simulink model "TaskServiceBase_FSM_revB"  (R2015b)
settings: Solver=ode4  StartTime=0.0  StopTime=inf  FixedStep=.01  RelTol=1e-3
settings Model: Creator=elliocm  LastModifiedBy=elliocm

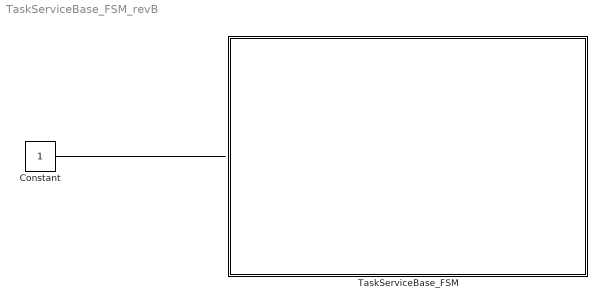
== system TaskServiceBase_FSM_revB ==
  Constant : Constant
  TaskServiceBase_FSM : Stateflow chart  RequirementInfo="{}  %GIDa_69d87331_3a4c_4800_b6a9_49c4bb62fd68"  TreatAsAtomicUnit=on
  wires:
  Constant/1 -> ?

== stateflow chart TaskServiceBase_FSM_revB/TaskServiceBase_FSM ==
  state Idle
    entry: state = 2
    state Idle_Request
      entry: SensorFootprintRequests_out = 0
    note: Simple Delay
        | (Consider Random Fail on TaskInit)
    state Idle_Success
      entry: SensorFootprintRequests_out = 1
    (default) -> Idle_Request
    Idle_Request -> (junction 51)
    (junction 51) -> Idle_Success : after(5,sec)
  state SensorRequest
    entry: state = 3
    state SensorRequest_Init
      entry: RouteRequest_out = 0
    note: Simple Delay
        | (Consider Random Fail on TaskInit)
    state SensorRequest_Success
      entry: RouteRequest_out = 1
    (default) -> SensorRequest_Init
    SensorRequest_Init -> (junction 64)
    (junction 64) -> SensorRequest_Success : after(3,sec)
  state Init
    entry: state = 1
    note: Simple Delay
        | (Consider Random Fail on TaskInit)
    state Init_Request
      entry: init_complete = 0
      TaskInitialized_out = 0
    state Init_Success
      entry: init_complete = 1
      TaskInitialized_out = 1
    (default) -> Init_Request
    Init_Request -> (junction 40)
    (junction 40) -> Init_Success : after(3,sec)
  state OptionRoutes
    entry: state = 4
    state OptionRoutes_Init
      entry: TaskPlanOptions_out = 0
    note: Simple Delay
        | (Consider Random Fail on TaskInit)
    state OptionRoutes_Success
      entry: TaskPlanOptions_out = 1
    (default) -> OptionRoutes_Init
    OptionRoutes_Init -> (junction 71)
    (junction 71) -> OptionRoutes_Success : after(10,sec)
  state Active
    entry: state = 8
    state Active_Init
      entry: TaskComplete_out = 0
    note: Simple Delay
        | (Consider Random Fail on TaskInit)
    state Active_Success
      entry: TaskComplete_out = 1
    (default) -> Active_Init
    Active_Init -> (junction 105)
    (junction 105) -> Active_Success : after(5,sec)
  state OptionSelected
    entry: state = 7
    state OptionSelected_Init
      entry: SensorFootprintRequests_out = 0
    note: Simple Delay
        | (Consider Random Fail on TaskInit)
    state OptionSelected_Success
      entry: SensorFootprintRequests_out = 1
    (default) -> OptionSelected_Init
    OptionSelected_Init -> (junction 97)
    (junction 97) -> OptionSelected_Success : after(5,sec)
  state OptionsPublished
    entry: state = 5
    state OptionsPublished_Init
      entry: RouteRequest_out = 0
    note: Simple Delay
        | (Consider Random Fail on TaskInit)
    state OptionsPublished_Success
      entry: RouteRequest_out = 1
    (default) -> OptionsPublished_Init
    OptionsPublished_Init -> (junction 80)
    (junction 80) -> OptionsPublished_Success : after(5,sec)
  state FinalRoutes
    entry: state = 6
    state FinalRoutes_Init
      entry: TaskImplementationResponse_out = 0
    note: Simple Delay
        | (Consider Random Fail on TaskInit)
    state FinalRoutes_Success
      entry: TaskImplementationResponse_out = 1
    (default) -> FinalRoutes_Init
    FinalRoutes_Init -> (junction 88)
    (junction 88) -> FinalRoutes_Success : after(5,sec)
  Init -> Idle : [init_complete && TaskInitialized_out]
  Idle -> SensorRequest : [SensorFootprintRequests_out]
  (default) -> Init
  OptionSelected -> SensorRequest [order 1] : [SensorFootprintRequests_out]
  SensorRequest -> OptionRoutes : [RouteRequest_out]
  Active -> Idle : [TaskComplete_out]
  OptionSelected -> Active [order 2]
  OptionRoutes -> OptionsPublished : [TaskPlanOptions_out]
  FinalRoutes -> OptionSelected : [TaskImplementationResponse_out]
  OptionsPublished -> FinalRoutes : [RouteRequest_out]
  data: state local; init_complete local; i local; TaskInitialized_out local; SensorFootprintRequests_out local; RouteRequest_out local; TaskPlanOptions_out local
